simulink model "main_sim_adapt_Gref_SP"  (Simulink 7.2)
settings: Solver=ode2  SolverMode=SingleTasking  StartTime=0.0  StopTime=tsim_max  FixedStep=dtsim  RelTol=1e-3
StopFcn:
  | %mkplt
values from neighbouring files (symbols this model uses):
  aero_surf_qbar_off = get_value('aero_surf_qbar_off')    [setup_claw.m]
  aero_surf_qbar_on = get_value('aero_surf_qbar_on')    [setup_claw.m]
  assertion_time = get_value('assertion_time')    [setup_sim.m]
  att_cmd_select = get_value('att_cmd_select')    [setup_sim.m]
  att_trim_IC = orientation.att'    [setup_claw.m]
  att_type_numbers = cell2mat(struct2cell(att_type))    [setup_constants.m]
  chi_trim_IC = orientation.Vchigam(2)    [setup_claw.m]
  command_time = engage_time + 2.0    [setup_sim.m]
  compute_all_rate_cols = get_value('compute_all_rate_cols')    [setup_claw.m]
  compute_all_vel_cols = get_value('compute_all_vel_cols')    [setup_claw.m]
  da_trim_IC = tmp(1)    [setup_claw.m]
  dc_L2W_IC = orientation.dc_L2W    [setup_claw.m]
  de_trim_IC = tmp(2)    [setup_claw.m]
  dr_trim_IC = tmp(3)    [setup_claw.m]
  dtsim = get_value('dtsim')    [setup_sim.m]
  E_trim_IC = MACH_pos_IC(2)    [setup_claw.m]
  Ed_trim_IC = MACH_vel_IC(2)    [setup_claw.m]
  gain_set = gain_set_next    (= 1)    [setup_claw.m]
  gain_var_struct = rmfield(gain_var_struct,setdiff(fieldnames(gain_var_struct),{'name','size'}))    [setup_claw.m]
  gamma_trim_IC = orientation.Vchigam(3)    [setup_claw.m]
  h_trim_IC = MACH_pos_IC(3)    [setup_claw.m]
  hd_trim_IC = MACH_vel_IC(3)    [setup_claw.m]
  ideal_vel_Kb = MACH_vel_Kb(1)    [setup_sim.m]
  MACH = rmfield(MACH,'vel_throt_lrlim')    [setup_claw.m]
  MACH_att_fb = get_value('MACH_att_fb','onerror',0)    [setup_claw.m]
  MACH_att_int_IC = (1-MACH_att_Kc).*MACH_quat_IC'    [setup_ideal.m]
  MACH_att_Kb = repval(att_kbnom,MACH.att_num_cv)    [setup_claw.m]
  MACH_att_Kc = Ki2Kc(MACH_att_Ki)    [setup_ideal.m]
  MACH_att_Ki = repval(att_fi,MACH.att_num_cv)    [setup_claw.m]
  MACH_gain_mat = vertcat(MACH_gain_mat, this_gain_mat)    [setup_claw.m]
  MACH_mass_IC = obac_params.mass_IC    [setup_claw.m]
  MACH_pos_IC = x_obac_IC(MACH.NEh_idx)    [setup_claw.m]
  MACH_pos_int_IC = (1-MACH_pos_Kc).*MACH_pos_IC' + MACH_vel_IC'./MACH_pos_Kb    [setup_ideal.m]
  MACH_pos_Kb = repval(pos_kbnom,MACH.pos_num_cv)    [setup_claw.m]
  MACH_pos_Kc = Ki2Kc(MACH_pos_Ki)    [setup_ideal.m]
  MACH_pos_Ki = repval(pos_fi,MACH.pos_num_cv)    [setup_claw.m]
  MACH_pqr_Bmat_IC = Bo(MACH.pqr_idx,MACH.pqr_u_idx)    [setup_claw.m]
  MACH_pqr_IC = pqr_trim_IC    [setup_claw.m]
  MACH_pqr_int_IC = (1-MACH_pqr_Kc).*MACH_pqr_IC'    [setup_ideal.m]
  MACH_pqr_Kb = repval(pqr_kbnom,MACH.pqr_num_cv)    [setup_claw.m]
  MACH_pqr_Kc = Ki2Kc(MACH_pqr_Ki)    [setup_ideal.m]
  MACH_pqr_Ki = repval(pqr_fi,MACH.pqr_num_cv)    [setup_claw.m]
  MACH_pqr_u_IC = [ vanes_trim_IC; tvc_trim_IC; rcs_trim_IC ]    [setup_claw.m]
  MACH_quat_IC = quat_trim_IC    [setup_claw.m]
  MACH_throttle_IC = throttle_trim_IC    [setup_claw.m]
  MACH_U_nom_IC = zeros(MACH.num_u,1)    [setup_claw.m]
  MACH_vel_Bmat_IC = MACH_vel_Bmat_IC*inv(vel_perts)    [setup_claw.m]
  MACH_vel_cvdnom_IC = repval(get_value('vel_cvdnom_IC','onerror',MACH_vel_cvdnom_IC),length(MACH_vel_cvdnom_IC))'    [setup_claw.m]
  MACH_vel_IC = orientation.NdEdhd'    [setup_claw.m]
  MACH_vel_int_IC = (1-MACH_vel_Kc).*MACH_vel_IC'    [setup_ideal.m]
  MACH_vel_Kb = repval(vel_kbnom,MACH.vel_num_cv)    [setup_claw.m]
  MACH_vel_Kc = Ki2Kc(MACH_vel_Ki)    [setup_ideal.m]
  MACH_vel_Ki = repval(vel_fi,MACH.vel_num_cv)    [setup_claw.m]
  MACH_vel_uold_IC = [ MACH_quat_IC; MACH_throttle_IC ]    [setup_claw.m]
  N_trim_IC = MACH_pos_IC(1)    [setup_claw.m]
  Nd_trim_IC = MACH_vel_IC(1)    [setup_claw.m]
  obac_params = define_model('obac', get_value('obac_model_type'))    [setup_claw.m]
  pos_cmd_select = get_value('pos_cmd_select')    [setup_sim.m]
  pqr_trim_IC = [ 0 0 0 ]'    [setup_claw.m]
  rate_cmd_select = get_value('rate_cmd_select')    [setup_sim.m]
  rcs_cvddes_thresh = get_value('rcs_cvddes_thresh')    [setup_claw.m]
  reset_camcmd_on_entry = get_value('reset_camcmd_on_entry')    [setup_claw.m]
  throttle_trim_IC = u_obac_IC(MACH.throttle_idx)    [setup_claw.m]
  trac_params = define_model('trac', get_value('trac_model_type','onerror',obac_params.model_type))    [setup_sim.m]
  use_auto_att_type = get_value('use_auto_att_type','onerror',0)    [setup_claw.m]
  use_eow_as_iv = get_value('use_eow_as_iv')    [setup_claw.m]
  use_full_surf_cmd = get_value('use_full_surf_cmd')    [setup_sim.m]
  use_nav = get_value('use_nav')    [setup_claw.m]
  use_NdEdh_pos = get_value('use_NdEdh_pos')    [setup_claw.m]
  use_pos_fltpath_lim = get_value('use_pos_fltpath_lim')    [setup_claw.m]
  use_throt_estimate = get_value('use_throt_estimate')    [setup_claw.m]
  use_variable_mass = get_value('use_variable_mass')    [setup_claw.m]
  use_wind_est = get_value('use_wind_est')    [setup_claw.m]
  V_trim_IC = orientation.Vchigam(1)    [setup_claw.m]
  vel_cmd_ramp_time = get_value('vel_cmd_ramp_time')    [setup_claw.m]
  vel_cmd_select = get_value('vel_cmd_select')    [setup_sim.m]
  x_trac_IC = x_obac_IC    [setup_sim.m]
undefined symbols (not defined in the file or in its folder): accel_cmd, alpha_trim, Am, att_type, B1, bb_ellipsoid, bb_params, Bm, C, constants, cosA, DiscIntNeverNeededParam, DZkx, DZtheta, E_rwy, Ed_cmd, eow_boundary, flag_autoadapt, flag_exsig, flag_uad, full_surf_llim, full_surf_ulim, gam_cmd_descent, gam_cmd_preflare, gamdot_cmd_descent, gamdot_cmd_flare, gamdot_cmd_preflare, Gamtheta, Gamx, hd_cmd, in_error_thresh, in_exsig_vecin, in_exsig_vecout, in_reset_stoptime, in_t_exsig, in_t_timer, in_tadaptoff_forced, in_tadapton_forced, Kb, Kxhat0, Kxnom, Kxstar, max_chi_cmd, max_LOS_rate, max_vel_cmd, min_chi_cmd, min_vel_cmd, modes, N_rwy, Nd_cmd, Nrbf, P, pos, Sig, sinA, target_pos_IC, target_range_blind, target_range_detect, target_range_homing, target_vel_IC ... (+11)
libraries: simulink x44, utility_lib x36, mach_lib x24, model_lib x13, simulink_need_slupdate x8, models x8
(part 8 of 8)

== system main_sim_adapt_Gref_SP/control input (modified)/control input/form control input/select command/pos cmd select/convert if use_Vchigam ==
  cmd_bus : Inport  OutDataType=sfix(16)  OutScaling=2^0
  Bus Assignment : BusAssignment  AssignedSignals=Nd_cmd,Ed_cmd
  Bus Selector3 : BusSelector  OutputSignals=Nd_cmd,Ed_cmd,att3_cmd,h_cmd  OutputAsBus=on
  Bus Selector5 : BusSelector  OutputSignals=V_cmd,chi_cmd,use_Vchigam
  Constant : Constant  Value=0  OutDataType=sfix(16)  OutScaling=2^0
  Switch : Switch  Threshold=0.5
  Terminator : Terminator
  vchigam2NdEdhd : utility_lib/vchigam2NdEdhd  SystemSampleTime=-1
  pos_cmd : Outport  OutDataType=sfix(16)  OutScaling=2^0
  wires:
  cmd_bus/1 -> Bus Selector5/1, Bus Selector3/1
  vchigam2NdEdhd/1 -> Bus Assignment/2
  vchigam2NdEdhd/2 -> Bus Assignment/3
  vchigam2NdEdhd/3 -> Terminator/1
  Bus Selector5/1 -> vchigam2NdEdhd/1  "<V_cmd>"
  Bus Selector3/1 -> Bus Assignment/1, Switch/3
  Bus Selector5/3 -> Switch/2  "<use_Vchigam>"
  Bus Assignment/1 -> Switch/1
  Switch/1 -> pos_cmd/1
  Bus Selector5/2 -> vchigam2NdEdhd/2  "<chi_cmd>"
  Constant/1 -> vchigam2NdEdhd/3

== system main_sim_adapt_Gref_SP/control input (modified)/control input/form control input/select command/vel cmd select/convert if use_Vchigam ==
  cmd_bus : Inport  OutDataType=sfix(16)  OutScaling=2^0
  Bus Assignment : BusAssignment  AssignedSignals=Nd_cmd,Ed_cmd,hd_cmd
  Bus Selector3 : BusSelector  OutputSignals=Nd_cmd,Ed_cmd,att3_cmd,hd_cmd  OutputAsBus=on
  Bus Selector5 : BusSelector  OutputSignals=V_cmd,chi_cmd,gamma_cmd,use_Vchigam
  Switch : Switch  Threshold=0.5
  vchigam2NdEdhd : utility_lib/vchigam2NdEdhd  SystemSampleTime=-1
  vel_cmd : Outport  OutDataType=sfix(16)  OutScaling=2^0
  wires:
  cmd_bus/1 -> Bus Selector5/1, Bus Selector3/1
  vchigam2NdEdhd/1 -> Bus Assignment/2
  vchigam2NdEdhd/2 -> Bus Assignment/3
  vchigam2NdEdhd/3 -> Bus Assignment/4
  Bus Selector5/1 -> vchigam2NdEdhd/1  "<V_cmd>"
  Bus Selector5/2 -> vchigam2NdEdhd/2  "<chi_cmd>"
  Bus Selector5/3 -> vchigam2NdEdhd/3  "<gamma_cmd>"
  Bus Selector3/1 -> Bus Assignment/1, Switch/3
  Bus Selector5/4 -> Switch/2  "<use_Vchigam>"
  Bus Assignment/1 -> Switch/1
  Switch/1 -> vel_cmd/1

== system main_sim_adapt_Gref_SP/control input (modified)/control input/generate commands/pos cmd generator/circle pos cmd/Ramp ==
  From Workspace1 : FromWorkspace  VariableName=[ 0 initial_output ; start_time initial_output ; start_time+1 initial_output+slope ]  SampleTime=MACH.dt
  ramp : Outport  OutDataType=sfix(16)  OutScaling=2^0
  wires:
  From Workspace1/1 -> ramp/1

== matlab function claw_main/rate_loops/allocation/RCS allocation/Embedded MATLAB Function ==
  data: Bmat input double; wght_cv input double; ulim input double; llim input double; cvd_des input double; rcs_cmd output double; minerr output double; scale output double; cvd_actual output double; err_thresh input double; rcs_use_in input double
function [rcs_cmd, minerr, scale, cvd_actual] = rcs_alloc(Bmat, wght_cv, ulim, llim, cvd_des, err_thresh, rcs_use_in)

rcs_quant = 0;
scale = 1;

nrcs = size(Bmat,2);


if(nrcs == 6)
    % assume fake RCS
    gang_pos = [0 0 0; 0 0 0; 1 1 0; 1 0 0; 0 0 1; 0 1 0];
    gang_neg = [1 1 0; 0 0 1; 0 0 0; 0 1 0; 0 0 0; 1 0 0];

    gain_factor = 1./diag(Bmat*gang_pos);
    rcs_cmd = gang_neg*(gain_factor.*max(0,-cvd_des)) + gang_pos*(gain_factor.*max(0,cvd_des));
    if(rcs_quant > 0)
        rcs_cmd = round(rcs_cmd/rcs_quant)*rcs_quant;
    end
    rcs_cmd = max(min(rcs_cmd,ulim),llim);
    cvd_actual = Bmat*rcs_cmd;
    minerr = norm_vec(cvd_actual - cvd_des);
    
    return
end

rcs_cmd = llim;
cvd_actual = Bmat*rcs_cmd; 
minerr = norm_vec((cvd_actual - cvd_des).*wght_cv);

if(minerr <= err_thresh)
    return
end

Bmat = diag(wght_cv)*Bmat;
cvd_des = wght_cv.*cvd_des;

scale_trial = 1;
normsq_cvd_trial = 0;

powersof2 = 2.^[0:nrcs-1];
bllim = uint32(powersof2*llim);
bulim = uint32(powersof2*ulim);
rcs_use_all = uint32([1:2^nrcs-1]');
rcs_use_tmp = bitor(rcs_use_all,uint32(bllim));
rcs_use_tmp = bitand(rcs_use_tmp,uint32(bulim));
rcs_use = rcs_use_in.*eq(rcs_use_tmp,rcs_use_all);

if(~any(rcs_use))
    return
end

for i = 1:length(rcs_use)
    
    if(~rcs_use(i))
        continue
    end
    
    rcson = double(bitget(uint32(i),1:nrcs))';
    cvd_trial = Bmat*rcson;
    
    % optional scaling
    if(0)
        scale_trial = dot(cvd_des,cvd_trial);
        if(scale_trial < 0)
            continue
        end
        
        normsq_cvd_trial = dot(cvd_trial,cvd_trial);
        if(normsq_cvd_trial <= scale_trial)
            scale_trial = 1;
        else
            scale_trial = dot(cvd_des,cvd_trial)/normsq_cvd_trial;
            cvd_trial = cvd_trial*scale_trial;
        end
    end
    
    cvd_ex = cvd_trial - cvd_des;
    err = norm_vec(cvd_ex);
    if(err < minerr)
        scale = scale_trial;
        rcs_cmd = rcson*scale;
        minerr = err;
        cvd_actual = cvd_trial./wght_cv;
    end
end

function out = norm_vec(in)

out = sqrt(sum(in.^2));

return

== matlab function claw_main/rate_loops/bangbang/Bang Bang ==
  data: bb_params input double; bb_ellipsoid input double; debug_output output double; cvddes output double; dir output double; use_bb output double; att_cvc input double; att_cv input double; timer output double; pqr input double; inertia input double; enable_bb input double; cvddes_lin input double; dir_old input double; use_bb_old input double; timer_old input double
function [debug_output,cvddes,dir,use_bb,timer] = bangbang(bb_params,bb_ellipsoid,att_cvc,att_cv,pqr,inertia,enable_bb,cvddes_lin,dir_old,use_bb_old,timer_old)
% This block supports an embeddable subset of the MATLAB language.
% See the help menu for details. 

dt = bb_params(1) ;
timer_max = bb_params(2) ;
att_thresh = bb_params(3) ;
rate_thresh = bb_params(4) ;
att_diff_thresh = bb_params(5) ;
pp_params = bb_params(6:end) ;

debug_output = zeros(12,1) ;
cvddes = cvddes_lin ;
use_bb = 0 ;
dir = zeros(3,1) ;
timer = timer_old ;

if( ~enable_bb )
    return
end
    
trans = qmpy([1 -1 -1 -1]'.*att_cv,att_cvc) ;

% default is to use dir_old if we were in bangbang last cycle,
% and the timer has not expired
use_dir_old = use_bb_old ;
if( use_dir_old )
    timer = timer + dt ;
    if( timer > timer_max )
        % if timer expires, don't use dir_old
        use_dir_old = 0 ;
    end
end

% compute att using current transformation quat
trans_mag = trans(1) ;
trans_dir = trans(2:4) ;
att = -2*atan2(norm_vec3(trans_dir),trans_mag) ;
att_old = -2*atan2(dir_old'*trans_dir,trans_mag) ;

% choose arbitrary att (and dir) sign to be the same as that computed using
% dir_old.  This is equivalent to making dir_old'*trans_dir positive.
if( att*att_old < 0 )
    att = -att ;
    trans_dir = -trans_dir ;
end

% if we intended to use dir_old, but the angle computed using
% dir_old is significantly different than that derived using the current
% transformation, we will use current dir.
% NOTE: the angle test below works only because att has been adjusted
% to have the same sign as att_old, and both result from atan2 
if( use_dir_old )
    if( abs(att - att_old) > att_diff_thresh )
        use_dir_old = 0 ;
    else
        dir = dir_old ;
        att = att_old ;
    end
end

% check condition to enter (or stay in) bangbang
if( abs(att) > att_thresh )
    use_bb = 1 ;
    
    if( ~use_dir_old )
        dir = trans_dir/norm_vec3(trans_dir) ;
        timer = 0 ;
    end

elseif( max(abs(pqr)) > rate_thresh )
    use_bb = 1 ;
    
    % if small attitude error, set dir based on rates
    if( ~use_dir_old )
        dir = pqr/norm_vec3(pqr) ;
        att = -2*atan2(dir'*trans_dir,trans_mag) ;
        timer = 0 ;
    end
else
    % even though not used, pass dir_old through for in case of ~use_bb
    dir = dir_old ;
    att = att_old ;
end

% Note: cvddes has been set to a default value of cvddes_lin

if( use_bb )
    rate = pqr'*dir ;
    accel_max = get_ellipsoid_scaling(inertia*dir,bb_ellipsoid) ;
    accel_min = -accel_max ;
    pp_params(1) = accel_max ;
    pp_params(2) = accel_min ;
    [outside,accel] = pp(pp_params,att,rate) ;
    
    if( outside <= 1 )
        % use default cvddes (cvddes_lin)
        use_bb = 0 ; 
    else
        % eliminate component of linear command in direction dir
        cvddes = cvddes - (dir'*cvddes)*dir ;
    end
else
    % use default cvddes (cvddes_lin)
    rate = 0 ;
    outside = 0 ;
    accel = 0 ;
end

% saturate command at ellipsoid
blend_lin_claw = cvddes*min(get_ellipsoid_scaling(inertia*cvddes,bb_ellipsoid),1) ;

% add component from bangbang
blend_bb_claw = accel*dir ;
cvddes = blend_lin_claw + blend_bb_claw ;

pp_utQu = 1/get_ellipsoid_scaling(inertia*cvddes,bb_ellipsoid) ;
debug_output = [att;att_old;rate;outside;accel;pp_utQu;blend_bb_claw;blend_lin_claw] ;

if( ~use_bb )
    
    % if not using bangbang reset the timer, and set dir to zero
    timer = 0 ;
    % dir used for cvd_des blending is now zeroed outside of this block,
    % so that dir can be retained through a temporary ~use_bb condition
%     dir = 0*dir ;
end

function r = qmpy(p,q)

p0 = p(1) ;
p1 = p(2) ;
p2 = p(3) ;
p3 = p(4) ;

q0 = q(1) ;
q1 = q(2) ;
q2 = q(3) ;
q3 = q(4) ;

r0 = p0 * q0 - p1 * q1 - p2 * q2 - p3 * q3 ;
r1 = p0 * q1 + p1 * q0 + p2 * q3 - p3 * q2 ;
r2 = p0 * q2 - p1 * q3 + p2 * q0 + p3 * q1 ;
r3 = p0 * q3 + p1 * q2 - p2 * q1 + p3 * q0 ;

r = [ r0 r1 r2 r3 ]' ;

function scale = get_ellipsoid_scaling(dir,ellipsoid)
    scale = 1/max(sqrt(dir'*(ellipsoid*dir)),1e-12) ;

function [outside,accel] = pp(params,att,rate)

% the linear control law is
% accel = ww^2 * ( att_cmd - att ) - 2 * zeta * ww * rate

amax = params(1) ; 
amin = params(2) ; 
ww = params(3) ;  
zeta = params(4) ; 
rate_des1 = params(5) ; 
rate_des2 = params(6) ;

% make switch curves conservative
swcurve_shrink = 1.0 ;

swcurve_pos = 0.5 * rate^2 - swcurve_shrink * amin * att ;
swcurve_neg = 0.5 * rate^2 - swcurve_shrink * amax * att ;

% replace ellipse with parallelogram
% outside = ( ww^2 * att^2 + 2 * zeta * ww * att * rate + rate^2 ) / ( ( 1 - zeta^2 ) * amax^2 / ww^2 ) ;
sx1 = 1 + zeta + 4 * zeta^2 ;
sv1 = -0.5 - 2 * zeta ;
sx2 = 1 - 4 * zeta^2
sv2 = 2 * zeta ;
p1 = [sx1; sv1] ;
p2 = [sx2; sv2] ;

outside = 2*ww/amax*max(abs(([p2+p1 p2-p1]\[att*ww; rate])))
accel = 0 ;

if( outside <= 1 )
    return
end

if( rate > 0 )
    if( swcurve_pos < 0 )
        if( rate < rate_des1 )
            accel = amax ;
        elseif( rate < rate_des2 )
            accel = 0 ;
        else
            accel = amin ;
        end
    else
        accel = amin ;
    end
else
    if( swcurve_neg < 0 )
        if( rate > -rate_des1 )
            accel = amin ;
        elseif( rate > - rate_des2 )
            accel = 0 ;
        else
            accel = amax ;
        end
    else
        accel = amax ;
    end
end


function out = norm_vec3(in)

out = sqrt(in(1)^2 + in(2)^2 + in(3)^2);

return
